simulink model "SistemaC"  (R2023a)
settings: Solver=ode23t  StartTime=0.0  StopTime=10  MaxStep=1E-3  RelTol=1e-3
libraries: fl_lib x21, nesl_utility x9, slpidlib x2
settings Model: LastModifiedBy=josu5
settings DataIOCC: ReturnWorkspaceOutputs=off  TimeSaveName=t
settings DebuggingCC: AlgebraicLoopMsg=none  ArtificialAlgebraicLoopMsg=none  MaxConsecutiveZCsMsg=none
settings RTWCC: GPUComputeCapability=5.0

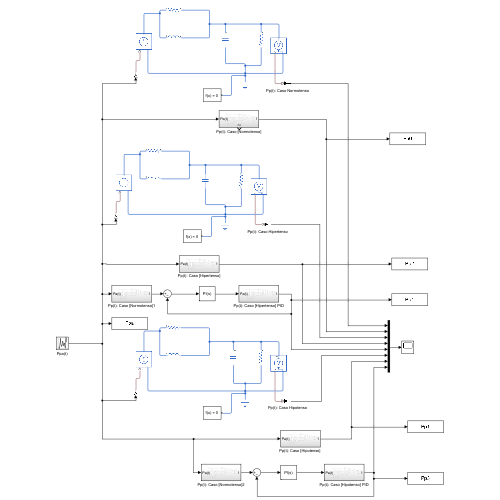
[thumbnail: Simulink's stored preview of the top-level diagram]
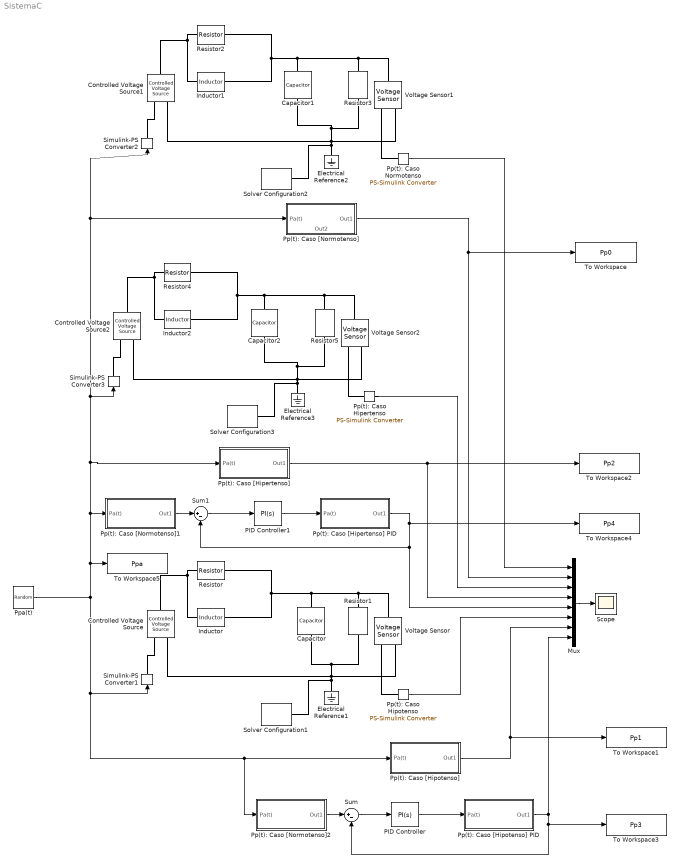
== system SistemaC ==
  Capacitor : fl_lib/Electrical/Electrical Elements/Capacitor  c=0.250 F  r=1e-6 Ohm  g=0 1/Ohm  i_specify=off  i_priority=None  i=0 A  i_nominal_specify=off  i_nominal_unit=A  i_nominal_value=1  v_specify=off  v_priority=None  v=0 V  v_nominal_specify=off  v_nominal_unit=V  v_nominal_value=1  vc_specify=off  vc_priority=High  vc=0 V  vc_nominal_specify=off  vc_nominal_unit=V  vc_nominal_value=1
  Capacitor1 : fl_lib/Electrical/Electrical Elements/Capacitor  c=1.5 F  r=1e-6 Ohm  g=0 1/Ohm  i_specify=off  i_priority=None  i=0 A  i_nominal_specify=off  i_nominal_unit=A  i_nominal_value=1  v_specify=off  v_priority=None  v=0 V  v_nominal_specify=off  v_nominal_unit=V  v_nominal_value=1  vc_specify=off  vc_priority=High  vc=0 V  vc_nominal_specify=off  vc_nominal_unit=V  vc_nominal_value=1
  Capacitor2 : fl_lib/Electrical/Electrical Elements/Capacitor  c=2.5 F  r=1e-6 Ohm  g=0 1/Ohm  i_specify=off  i_priority=None  i=0 A  i_nominal_specify=off  i_nominal_unit=A  i_nominal_value=1  v_specify=off  v_priority=None  v=0 V  v_nominal_specify=off  v_nominal_unit=V  v_nominal_value=1  vc_specify=off  vc_priority=High  vc=0 V  vc_nominal_specify=off  vc_nominal_unit=V  vc_nominal_value=1
  Controlled Voltage Source : fl_lib/Electrical/Electrical Sources/Controlled Voltage Source
  Controlled Voltage Source1 : fl_lib/Electrical/Electrical Sources/Controlled Voltage Source
  Controlled Voltage Source2 : fl_lib/Electrical/Electrical Sources/Controlled Voltage Source
  Electrical Reference1 : fl_lib/Electrical/Electrical Elements/Electrical Reference
  Electrical Reference2 : fl_lib/Electrical/Electrical Elements/Electrical Reference
  Electrical Reference3 : fl_lib/Electrical/Electrical Elements/Electrical Reference
  Inductor : fl_lib/Electrical/Electrical Elements/Inductor  l=0.005 H  r=0 Ohm  g=1e-9 1/Ohm  i_specify=off  i_priority=None  i=0 A  i_nominal_specify=off  i_nominal_unit=A  i_nominal_value=1  v_specify=off  v_priority=None  v=0 V  v_nominal_specify=off  v_nominal_unit=V  v_nominal_value=1  i_L_specify=off  i_L_priority=High  i_L=0 A  i_L_nominal_specify=off  i_L_nominal_unit=A  i_L_nominal_value=1
  Inductor1 : fl_lib/Electrical/Electrical Elements/Inductor  l=0.010 H  r=0 Ohm  g=1e-9 1/Ohm  i_specify=off  i_priority=None  i=0 A  i_nominal_specify=off  i_nominal_unit=A  i_nominal_value=1  v_specify=off  v_priority=None  v=0 V  v_nominal_specify=off  v_nominal_unit=V  v_nominal_value=1  i_L_specify=off  i_L_priority=High  i_L=0 A  i_L_nominal_specify=off  i_L_nominal_unit=A  i_L_nominal_value=1
  Inductor2 : fl_lib/Electrical/Electrical Elements/Inductor  l=0.020 H  r=0 Ohm  g=1e-9 1/Ohm  i_specify=off  i_priority=None  i=0 A  i_nominal_specify=off  i_nominal_unit=A  i_nominal_value=1  v_specify=off  v_priority=None  v=0 V  v_nominal_specify=off  v_nominal_unit=V  v_nominal_value=1  i_L_specify=off  i_L_priority=High  i_L=0 A  i_L_nominal_specify=off  i_L_nominal_unit=A  i_L_nominal_value=1
  Mux : Mux  Inputs=8
  PID Controller : slpidlib/PID Controller  Controller=PI  Form=Parallel  TimeDomain=Continuous-time  UseExternalTs=off  SampleTime=-1  IntegratorMethod=Forward Euler  FilterMethod=Forward Euler  ControllerParametersSource=internal  P=1.000340631088294622  I=404.434384377147  UseKiTs=off  D=0  N=100  UseFilter=on  TunerSelectOption=Transfer Function Based (PID Tuner App)  InitialConditionSource=internal  InitialConditionForIntegrator=0  InitialConditionForFilter=0  DifferentiatorICPrevScaledInput=0  ExternalReset=none  TrackingMode=off  Kt=1  LimitOutput=off  SatLimitsSource=internal  UpperSaturationLimit=inf  LowerSaturationLimit=-inf  LinearizeAsGain=on  AntiWindupMode=none  Kb=1  LimitIntegrator=off  UpperIntegratorSaturationLimit=inf  LowerIntegratorSaturationLimit=-inf  POutMin=[]  POutMax=[]  IOutMin=[]  IOutMax=[]  DOutMin=[]  DOutMax=[]  NOutMin=[]  NOutMax=[]  SumOutMin=[]  SumOutMax=[]  SaturationOutMin=[]  SaturationOutMax=[]  PParamMin=[]  PParamMax=[]  IParamMin=[]  IParamMax=[]  DParamMin=[]  DParamMax=[]  NParamMin=[]  NParamMax=[]  KbParamMin=[]  KbParamMax=[]  KtParamMin=[]  KtParamMax=[]  KbOutMin=[]  KbOutMax=[]  KtOutMin=[]  KtOutMax=[]  IntegratorOutMin=[]  IntegratorOutMax=[]  FilterOutMin=[]  FilterOutMax=[]  SumI1OutMin=[]  SumI1OutMax=[]  SumI2OutMin=[]  SumI2OutMax=[]  SumI3OutMin=[]  SumI3OutMax=[]  SumI4OutMin=[]  SumI4OutMax=[]  SumDOutMin=[]  SumDOutMax=[]  DifferentiatorOutMin=[]  DifferentiatorOutMax=[]  FilterDiffOutCoefMin=[]  FilterDiffOutCoefMax=[]  ReciprocalOutMin=[]  ReciprocalOutMax=[]  SumDenOutMin=[]  SumDenOutMax=[]  SumNumOutMin=[]  SumNumOutMax=[]  DivideOutMin=[]  DivideOutMax=[]  UdiffTsProdOutMin=[]  UdiffTsProdOutMax=[]  NTsProdOutMin=[]  NTsProdOutMax=[]  UintegralTsProdOutMin=[]  UintegralTsProdOutMax=[]  UngainTsProdOutMin=[]  UngainTsProdOutMax=[]  ClampingZeroOutDataTypeStr=Inherit: Inherit via back propagation  ClampingZeroOutMin=[]  ClampingZeroOutMax=[]  FilterDenConstantOutDataTypeStr=Inherit: Inherit via back propagation  FilterDenConstantOutMin=[]  FilterDenConstantOutMax=[]  PCopyOutDataTypeStr=Inherit: Inherit via back propagation  PCopyOutMin=[]  PCopyOutMax=[]  NCopyOutDataTypeStr=Inherit: Inherit via back propagation  NCopyOutMin=[]  NCopyOutMax=[]  IntegratorContinuousStateAttributes=''  IntegratorStateMustResolveToSignalObject=off  IntegratorRTWStateStorageClass=Auto  FilterContinuousStateAttributes=''  FilterStateMustResolveToSignalObject=off  FilterRTWStateStorageClass=Auto  ParallelPVariant=InternalParameters  IdealPVariant=Disabled  IVariant=InternalParameters  DVariant=Disabled  IntegratorVariant=Continuous  SatVariant=Disabled  AWVariant=Passthrough  PCopyVariant=Disabled  TRVariant=Disabled  FdbkBlocksVariant=Forward  IdealPFdbkVariant=Disabled  SatFdbkVariant=Disabled  DerivativeFilterVariant=Disabled  NVariant=Disabled  NCopyVariant=Disabled_SignalSpec  FilterICVariant=Disabled  IntegratorICVariant=InternalICs  ExternalResetVariant=Disabled  TRSumVariant=Passthrough  SumFdbkVariant=Disabled  SumVariant=Sum_PI  TsampFilterVariant=InternalTs  TsampNgainVariant=Passthrough  TsampIntegralVariant=Disabled_SignalSpec  ExternalSaturationOutDataTypeStr=Inherit: Same as second input
  PID Controller1 : slpidlib/PID Controller  Controller=PI  Form=Parallel  TimeDomain=Continuous-time  UseExternalTs=off  SampleTime=-1  IntegratorMethod=Forward Euler  FilterMethod=Forward Euler  ControllerParametersSource=internal  P=10  I=103.569197822789  UseKiTs=off  D=0  N=100  UseFilter=on  TunerSelectOption=Transfer Function Based (PID Tuner App)  InitialConditionSource=internal  InitialConditionForIntegrator=0  InitialConditionForFilter=0  DifferentiatorICPrevScaledInput=0  ExternalReset=none  TrackingMode=off  Kt=1  LimitOutput=off  SatLimitsSource=internal  UpperSaturationLimit=inf  LowerSaturationLimit=-inf  LinearizeAsGain=on  AntiWindupMode=none  Kb=1  LimitIntegrator=off  UpperIntegratorSaturationLimit=inf  LowerIntegratorSaturationLimit=-inf  POutMin=[]  POutMax=[]  IOutMin=[]  IOutMax=[]  DOutMin=[]  DOutMax=[]  NOutMin=[]  NOutMax=[]  SumOutMin=[]  SumOutMax=[]  SaturationOutMin=[]  SaturationOutMax=[]  PParamMin=[]  PParamMax=[]  IParamMin=[]  IParamMax=[]  DParamMin=[]  DParamMax=[]  NParamMin=[]  NParamMax=[]  KbParamMin=[]  KbParamMax=[]  KtParamMin=[]  KtParamMax=[]  KbOutMin=[]  KbOutMax=[]  KtOutMin=[]  KtOutMax=[]  IntegratorOutMin=[]  IntegratorOutMax=[]  FilterOutMin=[]  FilterOutMax=[]  SumI1OutMin=[]  SumI1OutMax=[]  SumI2OutMin=[]  SumI2OutMax=[]  SumI3OutMin=[]  SumI3OutMax=[]  SumI4OutMin=[]  SumI4OutMax=[]  SumDOutMin=[]  SumDOutMax=[]  DifferentiatorOutMin=[]  DifferentiatorOutMax=[]  FilterDiffOutCoefMin=[]  FilterDiffOutCoefMax=[]  ReciprocalOutMin=[]  ReciprocalOutMax=[]  SumDenOutMin=[]  SumDenOutMax=[]  SumNumOutMin=[]  SumNumOutMax=[]  DivideOutMin=[]  DivideOutMax=[]  UdiffTsProdOutMin=[]  UdiffTsProdOutMax=[]  NTsProdOutMin=[]  NTsProdOutMax=[]  UintegralTsProdOutMin=[]  UintegralTsProdOutMax=[]  UngainTsProdOutMin=[]  UngainTsProdOutMax=[]  ClampingZeroOutDataTypeStr=Inherit: Inherit via back propagation  ClampingZeroOutMin=[]  ClampingZeroOutMax=[]  FilterDenConstantOutDataTypeStr=Inherit: Inherit via back propagation  FilterDenConstantOutMin=[]  FilterDenConstantOutMax=[]  PCopyOutDataTypeStr=Inherit: Inherit via back propagation  PCopyOutMin=[]  PCopyOutMax=[]  NCopyOutDataTypeStr=Inherit: Inherit via back propagation  NCopyOutMin=[]  NCopyOutMax=[]  IntegratorContinuousStateAttributes=''  IntegratorStateMustResolveToSignalObject=off  IntegratorRTWStateStorageClass=Auto  FilterContinuousStateAttributes=''  FilterStateMustResolveToSignalObject=off  FilterRTWStateStorageClass=Auto  ParallelPVariant=InternalParameters  IdealPVariant=Disabled  IVariant=InternalParameters  DVariant=Disabled  IntegratorVariant=Continuous  SatVariant=Disabled  AWVariant=Passthrough  PCopyVariant=Disabled  TRVariant=Disabled  FdbkBlocksVariant=Forward  IdealPFdbkVariant=Disabled  SatFdbkVariant=Disabled  DerivativeFilterVariant=Disabled  NVariant=Disabled  NCopyVariant=Disabled_SignalSpec  FilterICVariant=Disabled  IntegratorICVariant=InternalICs  ExternalResetVariant=Disabled  TRSumVariant=Passthrough  SumFdbkVariant=Disabled  SumVariant=Sum_PI  TsampFilterVariant=InternalTs  TsampNgainVariant=Passthrough  TsampIntegralVariant=Disabled_SignalSpec  ExternalSaturationOutDataTypeStr=Inherit: Same as second input
  Pp(t): Caso Hipertenso : nesl_utility/PS-Simulink Converter  PhysicalDomain=network_engine_domain  SubClassName=ps_output  LeftPortType=input  RightPortType=output  PseudoPeriodic=off  Frequencies=[]  VectorFormat=1-D array  Unit=inherit  AffineConversion=off
  Pp(t): Caso Hipotenso : nesl_utility/PS-Simulink Converter  PhysicalDomain=network_engine_domain  SubClassName=ps_output  LeftPortType=input  RightPortType=output  PseudoPeriodic=off  Frequencies=[]  VectorFormat=1-D array  Unit=inherit  AffineConversion=off
  Pp(t): Caso Normotenso : nesl_utility/PS-Simulink Converter  PhysicalDomain=network_engine_domain  SubClassName=ps_output  LeftPortType=input  RightPortType=output  PseudoPeriodic=off  Frequencies=[]  VectorFormat=1-D array  Unit=inherit  AffineConversion=off
  Pp(t): Caso [Hipertenso] : Subsystem
  Pp(t): Caso [Hipertenso] PID : Subsystem
  "Pp(t): Caso [Hipotenso] " : Subsystem
  Pp(t): Caso [Hipotenso] PID : Subsystem
  Pp(t): Caso [Normotenso] : Subsystem
      settings: PortSchema="{\"entries\":[{\"content\":{\"sides\":[{\"content\":{\"connectorIds\":[\"In1\"]},\"type\":\"ConnectorPlacement.EquallySpacedRectSide\",\"uuid\":\"31d49f5b-ec0b-4ba9-8ce0-c312c27acef8\"},{\"content\":{\"connectorIds\":[\"Out1\"],\"side\":\"RIGHT\"},\"type\":\"ConnectorPlacement.EquallySpacedRectSide\",\"uuid\":\"62992713-140b-4123-82a3-4e8e6168027d\"},{\"content\":{\"side\":\"TOP\"},\"type\":\"ConnectorPlacement.EquallySpacedRectSide\",\"uuid\":\"6cf9fc40-2f75-4534-a9ff-367cf75ce896\"},{\"content\":{\"connectorIds\":[\"Out2\"],\"side\":\"BOTTOM\"},\"type\":\"ConnectorPlacement.EquallySpacedRectSide\",\"uuid\":\"311e03a3-df68-4c99-90aa-93326344dd84\"}]},\"type\":\"ConnectorPlacement.EquallySpacedConnector\",\"uuid\":\"5b112b4e-a5b3-4dba-9e47-3b0de052d796\"}],\"packageUris\":[\"http://schema.mathworks.com/mf0/Connector/R2020b\"],\"version\":\"1.0\"}"
  Pp(t): Caso [Normotenso]1 : Subsystem
  Pp(t): Caso [Normotenso]2 : Subsystem
  Ppa(t) : UniformRandomNumber  Minimum=-0.2  Seed=106  SampleTime=0.5
  Resistor : fl_lib/Electrical/Electrical Elements/Resistor  R=0.020 Ohm  i_specify=off  i_priority=None  i=0 A  i_nominal_specify=off  i_nominal_unit=A  i_nominal_value=1  v_specify=off  v_priority=None  v=0 V  v_nominal_specify=off  v_nominal_unit=V  v_nominal_value=1
  Resistor1 : fl_lib/Electrical/Electrical Elements/Resistor  R=0.600 Ohm  i_specify=off  i_priority=None  i=0 A  i_nominal_specify=off  i_nominal_unit=A  i_nominal_value=1  v_specify=off  v_priority=None  v=0 V  v_nominal_specify=off  v_nominal_unit=V  v_nominal_value=1
  Resistor2 : fl_lib/Electrical/Electrical Elements/Resistor  R=0.033 Ohm  i_specify=off  i_priority=None  i=0 A  i_nominal_specify=off  i_nominal_unit=A  i_nominal_value=1  v_specify=off  v_priority=None  v=0 V  v_nominal_specify=off  v_nominal_unit=V  v_nominal_value=1
  Resistor3 : fl_lib/Electrical/Electrical Elements/Resistor  R=0.950 Ohm  i_specify=off  i_priority=None  i=0 A  i_nominal_specify=off  i_nominal_unit=A  i_nominal_value=1  v_specify=off  v_priority=None  v=0 V  v_nominal_specify=off  v_nominal_unit=V  v_nominal_value=1
  Resistor4 : fl_lib/Electrical/Electrical Elements/Resistor  R=0.050 Ohm  i_specify=off  i_priority=None  i=0 A  i_nominal_specify=off  i_nominal_unit=A  i_nominal_value=1  v_specify=off  v_priority=None  v=0 V  v_nominal_specify=off  v_nominal_unit=V  v_nominal_value=1
  Resistor5 : fl_lib/Electrical/Electrical Elements/Resistor  R=1.4 Ohm  i_specify=off  i_priority=None  i=0 A  i_nominal_specify=off  i_nominal_unit=A  i_nominal_value=1  v_specify=off  v_priority=None  v=0 V  v_nominal_specify=off  v_nominal_unit=V  v_nominal_value=1
  Scope : Scope
  Simulink-PS Converter1 : nesl_utility/Simulink-PS Converter  PhysicalDomain=network_engine_domain  SubClassName=ps_input  LeftPortType=input  RightPortType=output  PseudoPeriodic=off  Frequencies=[]  NoiseDistribution=none  NoiseParameters=[]  Unit=1  AffineConversion=off  FilteringAndDerivatives=provide  SimscapeFilterOrder=1  InputFilterTimeConstant=0.001  UdotUserProvided=0
  Simulink-PS Converter2 : nesl_utility/Simulink-PS Converter  PhysicalDomain=network_engine_domain  SubClassName=ps_input  LeftPortType=input  RightPortType=output  PseudoPeriodic=off  Frequencies=[]  NoiseDistribution=none  NoiseParameters=[]  Unit=1  AffineConversion=off  FilteringAndDerivatives=provide  SimscapeFilterOrder=1  InputFilterTimeConstant=0.001  UdotUserProvided=0
  Simulink-PS Converter3 : nesl_utility/Simulink-PS Converter  PhysicalDomain=network_engine_domain  SubClassName=ps_input  LeftPortType=input  RightPortType=output  PseudoPeriodic=off  Frequencies=[]  NoiseDistribution=none  NoiseParameters=[]  Unit=1  AffineConversion=off  FilteringAndDerivatives=provide  SimscapeFilterOrder=1  InputFilterTimeConstant=0.001  UdotUserProvided=0
  Solver Configuration1 : nesl_utility/Solver Configuration  PhysicalDomain=network_engine_domain  SubClassName=solver  LeftPortType=input  RightPortType=generic  Tones=[]  Harmonics=[]  SimulateNoise=off  Profile=off  UseLocalSampling=off  EnableSwitchedLinearOptims=on  FrequencyDomain=off  UseCCode=off  RelTol=0.001  AbsTol=0.001  MinStep=1e-09  ToWorkspace=off  RevertToSquareIcSolve=off  NumHomotopyIterations=100  PhasorMode=off  PhasorModeNumHarmonics=1  ConsistencySolver=NEWTON_XTOL_AFTER_FTOL  IndexReductionMethod=DerivativeReplacement  DoDC=off  ResidualTolerance=1e-09  ConsistencyTolSource=GLOBAL  ConsistencyAbsTol=0.001  ConsistencyRelTol=0.001  ConsistencyTolFactor=0.001  UseLocalSolver=off  LocalSolverChoice=NE_BACKWARD_EULER_ADVANCER  ResolveIndetEquations=on  FunctionEvalNumThread=1  LocalSolverSampleTime=0.001  DoFixedCost=off  MaxNonlinIter=3  MaxModeIter=2  ComputeImpulses=off  ImpulseIterations=2  LinearAlgebra=auto  LinearAlgebraNumThread=0  EquationFormulation=NE_TIME_EF  DelaysMemoryBudget=1024  AutomaticFiltering=on  FilteringTimeConstant=0.001  PartitionStorageMethod=AS_NEEDED  PartitionMemoryBudget=1024  PartitionMethod=ROBUST
  Solver Configuration2 : nesl_utility/Solver Configuration  PhysicalDomain=network_engine_domain  SubClassName=solver  LeftPortType=input  RightPortType=generic  Tones=[]  Harmonics=[]  SimulateNoise=off  Profile=off  UseLocalSampling=off  EnableSwitchedLinearOptims=on  FrequencyDomain=off  UseCCode=off  RelTol=0.001  AbsTol=0.001  MinStep=1e-09  ToWorkspace=off  RevertToSquareIcSolve=off  NumHomotopyIterations=100  PhasorMode=off  PhasorModeNumHarmonics=1  ConsistencySolver=NEWTON_XTOL_AFTER_FTOL  IndexReductionMethod=DerivativeReplacement  DoDC=off  ResidualTolerance=1e-09  ConsistencyTolSource=GLOBAL  ConsistencyAbsTol=0.001  ConsistencyRelTol=0.001  ConsistencyTolFactor=0.001  UseLocalSolver=off  LocalSolverChoice=NE_BACKWARD_EULER_ADVANCER  ResolveIndetEquations=on  FunctionEvalNumThread=1  LocalSolverSampleTime=0.001  DoFixedCost=off  MaxNonlinIter=3  MaxModeIter=2  ComputeImpulses=off  ImpulseIterations=2  LinearAlgebra=auto  LinearAlgebraNumThread=0  EquationFormulation=NE_TIME_EF  DelaysMemoryBudget=1024  AutomaticFiltering=on  FilteringTimeConstant=0.001  PartitionStorageMethod=AS_NEEDED  PartitionMemoryBudget=1024  PartitionMethod=ROBUST
  Solver Configuration3 : nesl_utility/Solver Configuration  PhysicalDomain=network_engine_domain  SubClassName=solver  LeftPortType=input  RightPortType=generic  Tones=[]  Harmonics=[]  SimulateNoise=off  Profile=off  UseLocalSampling=off  EnableSwitchedLinearOptims=on  FrequencyDomain=off  UseCCode=off  RelTol=0.001  AbsTol=0.001  MinStep=1e-09  ToWorkspace=off  RevertToSquareIcSolve=off  NumHomotopyIterations=100  PhasorMode=off  PhasorModeNumHarmonics=1  ConsistencySolver=NEWTON_XTOL_AFTER_FTOL  IndexReductionMethod=DerivativeReplacement  DoDC=off  ResidualTolerance=1e-09  ConsistencyTolSource=GLOBAL  ConsistencyAbsTol=0.001  ConsistencyRelTol=0.001  ConsistencyTolFactor=0.001  UseLocalSolver=off  LocalSolverChoice=NE_BACKWARD_EULER_ADVANCER  ResolveIndetEquations=on  FunctionEvalNumThread=1  LocalSolverSampleTime=0.001  DoFixedCost=off  MaxNonlinIter=3  MaxModeIter=2  ComputeImpulses=off  ImpulseIterations=2  LinearAlgebra=auto  LinearAlgebraNumThread=0  EquationFormulation=NE_TIME_EF  DelaysMemoryBudget=1024  AutomaticFiltering=on  FilteringTimeConstant=0.001  PartitionStorageMethod=AS_NEEDED  PartitionMemoryBudget=1024  PartitionMethod=ROBUST
  Sum : Sum  Inputs=|+-
  Sum1 : Sum  Inputs=|+-
  To Workspace : ToWorkspace  VariableName=Pp0  SampleTime=-1
  To Workspace1 : ToWorkspace  VariableName=Pp1  SampleTime=-1
  To Workspace2 : ToWorkspace  VariableName=Pp2  SampleTime=-1
  To Workspace3 : ToWorkspace  VariableName=Pp3  SampleTime=-1
  To Workspace4 : ToWorkspace  VariableName=Pp4  SampleTime=-1
  To Workspace5 : ToWorkspace  VariableName=Ppa  SampleTime=-1
  Voltage Sensor : fl_lib/Electrical/Electrical Sensors/Voltage Sensor
  Voltage Sensor1 : fl_lib/Electrical/Electrical Sensors/Voltage Sensor
  Voltage Sensor2 : fl_lib/Electrical/Electrical Sensors/Voltage Sensor
  wires:
  Ppa(t)/1 -> To Workspace5/1, Pp(t): Caso [Normotenso]1/1(Pa(t)), Pp(t): Caso [Hipertenso]/1(Pa(t)), Pp(t): Caso [Normotenso]/1(Pa(t)), Simulink-PS Converter2/1, Simulink-PS Converter3/1, Simulink-PS Converter1/1, "Pp(t): Caso [Hipotenso] "/1(Pa(t)), Pp(t): Caso [Normotenso]2/1(Pa(t))
  Mux/1 -> Scope/1
  Pp(t): Caso [Hipotenso] PID/1(Out1) -> Mux/8, To Workspace3/1, Sum/2
  Pp(t): Caso [Normotenso]2/1(Out1) -> Sum/1
  Pp(t): Caso [Normotenso]1/1(Out1) -> Sum1/1
  "Pp(t): Caso [Hipotenso] "/1(Out1) -> Mux/7, To Workspace1/1
  Pp(t): Caso Hipotenso/1 -> Mux/6
  Pp(t): Caso Hipertenso/1 -> Mux/3
  Pp(t): Caso Normotenso/1 -> Mux/1
  Pp(t): Caso [Normotenso]/1(Out1) -> Mux/2, To Workspace/1
  Sum/1 -> PID Controller/1
  PID Controller/1 -> Pp(t): Caso [Hipotenso] PID/1(Pa(t))
  Pp(t): Caso [Hipertenso]/1(Out1) -> To Workspace2/1, Mux/4
  Pp(t): Caso [Hipertenso] PID/1(Out1) -> Mux/5, Sum1/2, To Workspace4/1
  Sum1/1 -> PID Controller1/1
  PID Controller1/1 -> Pp(t): Caso [Hipertenso] PID/1(Pa(t))
  connections:
  Resistor/LConn1 -- Controlled Voltage Source/LConn1 -- Inductor/LConn1
  Resistor/RConn1 -- Inductor/RConn1 -- Voltage Sensor/LConn1 -- Resistor1/LConn1 -- Capacitor/LConn1
  Resistor1/RConn1 -- Solver Configuration1/RConn1 -- Electrical Reference1/LConn1 -- Voltage Sensor/RConn2 -- Controlled Voltage Source/RConn2 -- Capacitor/RConn1
  Simulink-PS Converter1/RConn1 -- Controlled Voltage Source/RConn1
  Voltage Sensor/RConn1 -- Pp(t): Caso Hipotenso/LConn1
  Resistor3/LConn1 -- Resistor2/RConn1 -- Inductor1/RConn1 -- Capacitor1/LConn1 -- Voltage Sensor1/LConn1
  Electrical Reference2/LConn1 -- Resistor3/RConn1 -- Capacitor1/RConn1 -- Voltage Sensor1/RConn2 -- Controlled Voltage Source1/RConn2 -- Solver Configuration2/RConn1
  Inductor1/LConn1 -- Resistor2/LConn1 -- Controlled Voltage Source1/LConn1
  Voltage Sensor1/RConn1 -- Pp(t): Caso Normotenso/LConn1
  Simulink-PS Converter2/RConn1 -- Controlled Voltage Source1/RConn1
  Inductor2/LConn1 -- Resistor4/LConn1 -- Controlled Voltage Source2/LConn1
  Electrical Reference3/LConn1 -- Solver Configuration3/RConn1 -- Voltage Sensor2/RConn2 -- Controlled Voltage Source2/RConn2 -- Resistor5/RConn1 -- Capacitor2/RConn1
  Resistor5/LConn1 -- Resistor4/RConn1 -- Inductor2/RConn1 -- Capacitor2/LConn1 -- Voltage Sensor2/LConn1
  Voltage Sensor2/RConn1 -- Pp(t): Caso Hipertenso/LConn1
  Simulink-PS Converter3/RConn1 -- Controlled Voltage Source2/RConn1

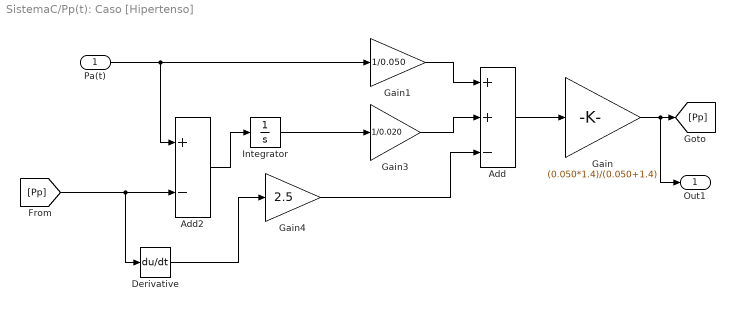
== system SistemaC/Pp(t): Caso [Hipertenso] ==
  Pa(t) : Inport
  Add : Sum  Inputs=++-
  Add2 : Sum  Inputs=+-
  Derivative : Derivative
  Gain : Gain  Gain=(0.050*1.4)/(0.050+1.4)
  Gain1 : Gain  Gain=1/0.050
  Gain3 : Gain  Gain=1/0.020
  Gain4 : Gain  Gain=2.5
  Integrator : Integrator
  Out1 : Outport
  wires:
  Add/1 -> Gain/1
  Pa(t)/1 -> Add2/1, Gain1/1
  Gain1/1 -> Add/1
  Gain3/1 -> Add/2
  Integrator/1 -> Gain3/1
  Add2/1 -> Integrator/1
  [Pp] -> Derivative/1, Add2/2
  Derivative/1 -> Gain4/1
  Gain4/1 -> Add/3
  Gain/1 -> Out1/1, [Pp]

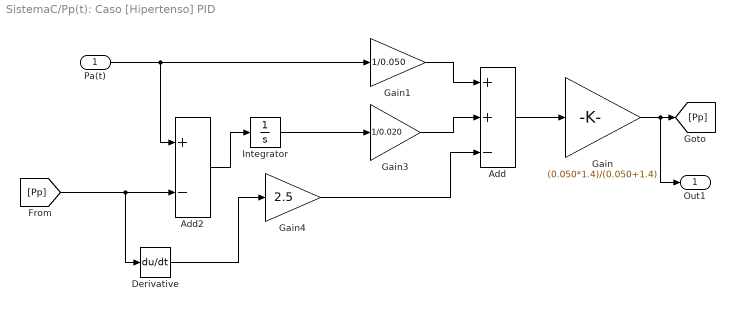
== system SistemaC/Pp(t): Caso [Hipertenso] PID ==
  Pa(t) : Inport
  Add : Sum  Inputs=++-
  Add2 : Sum  Inputs=+-
  Derivative : Derivative
  Gain : Gain  Gain=(0.050*1.4)/(0.050+1.4)
  Gain1 : Gain  Gain=1/0.050
  Gain3 : Gain  Gain=1/0.020
  Gain4 : Gain  Gain=2.5
  Integrator : Integrator
  Out1 : Outport
  wires:
  Add/1 -> Gain/1
  Pa(t)/1 -> Add2/1, Gain1/1
  Gain1/1 -> Add/1
  Gain3/1 -> Add/2
  Integrator/1 -> Gain3/1
  Add2/1 -> Integrator/1
  [Pp] -> Derivative/1, Add2/2
  Derivative/1 -> Gain4/1
  Gain4/1 -> Add/3
  Gain/1 -> Out1/1, [Pp]

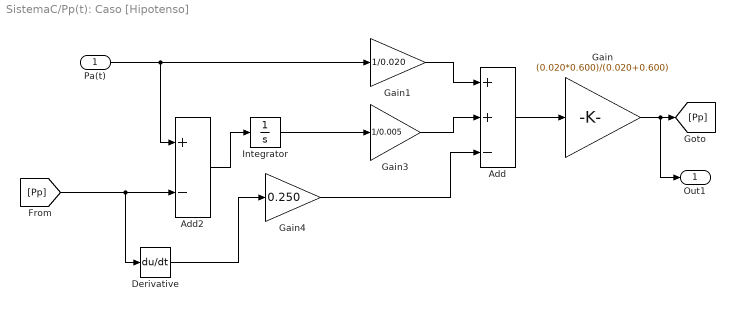
== system SistemaC/Pp(t): Caso [Hipotenso]  ==
  Pa(t) : Inport
  Add : Sum  Inputs=++-
  Add2 : Sum  Inputs=+-
  Derivative : Derivative
  Gain : Gain  Gain=(0.020*0.600)/(0.020+0.600)
  Gain1 : Gain  Gain=1/0.020
  Gain3 : Gain  Gain=1/0.005
  Gain4 : Gain  Gain=0.250
  Integrator : Integrator
  Out1 : Outport
  wires:
  Add/1 -> Gain/1
  Pa(t)/1 -> Add2/1, Gain1/1
  Gain1/1 -> Add/1
  Gain3/1 -> Add/2
  Integrator/1 -> Gain3/1
  Add2/1 -> Integrator/1
  [Pp] -> Derivative/1, Add2/2
  Derivative/1 -> Gain4/1
  Gain4/1 -> Add/3
  Gain/1 -> Out1/1, [Pp]

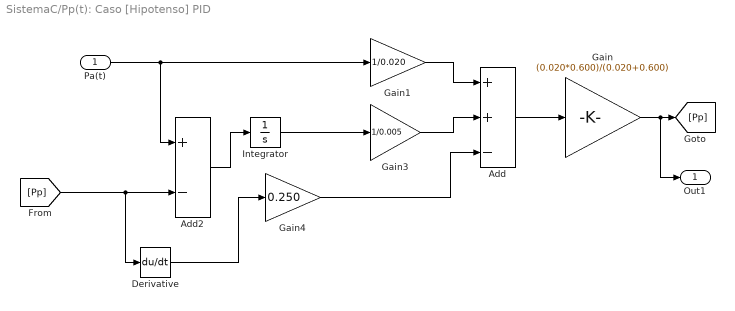
== system SistemaC/Pp(t): Caso [Hipotenso] PID ==
  Pa(t) : Inport
  Add : Sum  Inputs=++-
  Add2 : Sum  Inputs=+-
  Derivative : Derivative
  Gain : Gain  Gain=(0.020*0.600)/(0.020+0.600)
  Gain1 : Gain  Gain=1/0.020
  Gain3 : Gain  Gain=1/0.005
  Gain4 : Gain  Gain=0.250
  Integrator : Integrator
  Out1 : Outport
  wires:
  Add/1 -> Gain/1
  Pa(t)/1 -> Add2/1, Gain1/1
  Gain1/1 -> Add/1
  Gain3/1 -> Add/2
  Integrator/1 -> Gain3/1
  Add2/1 -> Integrator/1
  [Pp] -> Derivative/1, Add2/2
  Derivative/1 -> Gain4/1
  Gain4/1 -> Add/3
  Gain/1 -> Out1/1, [Pp]

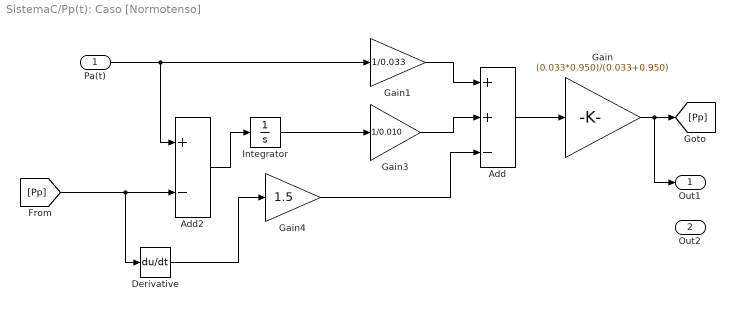
== system SistemaC/Pp(t): Caso [Normotenso] ==
  Pa(t) : Inport
  Add : Sum  Inputs=++-
  Add2 : Sum  Inputs=+-
  Derivative : Derivative
  Gain : Gain  Gain=(0.033*0.950)/(0.033+0.950)
  Gain1 : Gain  Gain=1/0.033
  Gain3 : Gain  Gain=1/0.010
  Gain4 : Gain  Gain=1.5
  Integrator : Integrator
  Out1 : Outport
  Out2 : Outport  Port=2
  wires:
  Add/1 -> Gain/1
  Pa(t)/1 -> Add2/1, Gain1/1
  Gain1/1 -> Add/1
  Gain3/1 -> Add/2
  Integrator/1 -> Gain3/1
  Add2/1 -> Integrator/1
  [Pp] -> Derivative/1, Add2/2
  Derivative/1 -> Gain4/1
  Gain4/1 -> Add/3
  Gain/1 -> Out1/1, [Pp]

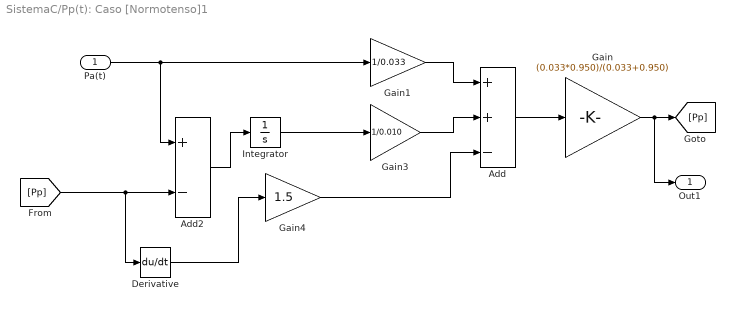
== system SistemaC/Pp(t): Caso [Normotenso]1 ==
  Pa(t) : Inport
  Add : Sum  Inputs=++-
  Add2 : Sum  Inputs=+-
  Derivative : Derivative
  Gain : Gain  Gain=(0.033*0.950)/(0.033+0.950)
  Gain1 : Gain  Gain=1/0.033
  Gain3 : Gain  Gain=1/0.010
  Gain4 : Gain  Gain=1.5
  Integrator : Integrator
  Out1 : Outport
  wires:
  Add/1 -> Gain/1
  Pa(t)/1 -> Add2/1, Gain1/1
  Gain1/1 -> Add/1
  Gain3/1 -> Add/2
  Integrator/1 -> Gain3/1
  Add2/1 -> Integrator/1
  [Pp] -> Derivative/1, Add2/2
  Derivative/1 -> Gain4/1
  Gain4/1 -> Add/3
  Gain/1 -> Out1/1, [Pp]

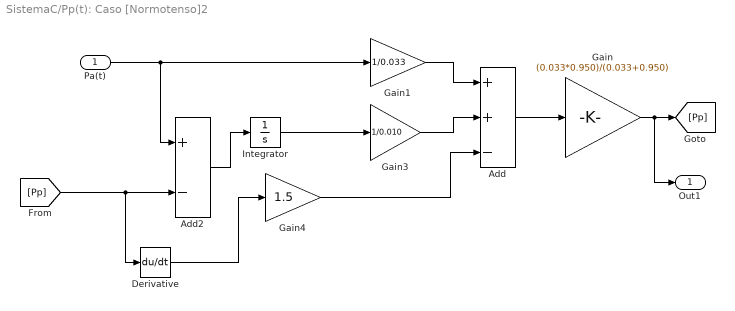
== system SistemaC/Pp(t): Caso [Normotenso]2 ==
  Pa(t) : Inport
  Add : Sum  Inputs=++-
  Add2 : Sum  Inputs=+-
  Derivative : Derivative
  Gain : Gain  Gain=(0.033*0.950)/(0.033+0.950)
  Gain1 : Gain  Gain=1/0.033
  Gain3 : Gain  Gain=1/0.010
  Gain4 : Gain  Gain=1.5
  Integrator : Integrator
  Out1 : Outport
  wires:
  Add/1 -> Gain/1
  Pa(t)/1 -> Add2/1, Gain1/1
  Gain1/1 -> Add/1
  Gain3/1 -> Add/2
  Integrator/1 -> Gain3/1
  Add2/1 -> Integrator/1
  [Pp] -> Derivative/1, Add2/2
  Derivative/1 -> Gain4/1
  Gain4/1 -> Add/3
  Gain/1 -> Out1/1, [Pp]
